simulink model "RaspberryPiMotorTest"  (R2023b)
settings: Solver=VariableStepAuto  StartTime=0.0  StopTime=10.0  RelTol=1e-3
libraries: raspberrypiBasiclib x3
settings Model: Creator=reedv  LastModifiedBy=reedv

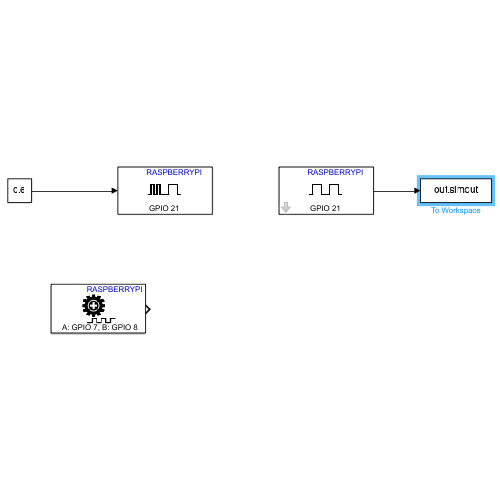
[thumbnail: Simulink's stored preview of the top-level diagram]
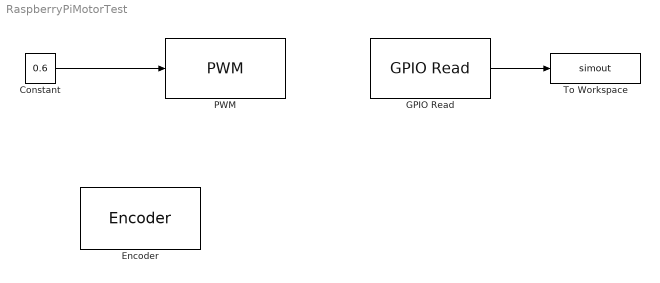
== system RaspberryPiMotorTest ==
  Constant : Constant  Value=0.6
  Encoder : raspberrypiBasiclib/Encoder  BoardProperty=Pi 4 Model B  InputA=GPIO 7  InputB=GPIO 8  Mode=No reset  SampleTime=-1
  GPIO Read : raspberrypiBasiclib/GPIO Read  board=Pi 4 Model B  gpio=21  internalResistor=Off  sampleTime=0.1  direction=Input  blockPlatform=Raspberry Pi
  PWM : raspberrypiBasiclib/PWM  board=Pi 2 Model B  Pin_=21  Frequency=50  blockPlatform=Raspberry Pi
  To Workspace : ToWorkspace  VariableName=simout  SaveFormat=Timeseries  SampleTime=-1
  wires:
  GPIO Read/1 -> To Workspace/1
  Constant/1 -> PWM/1
